simulink model "mseExampleDelayWithLoop"  (R2023b)
settings: Solver=VariableStepAuto  StartTime=0.0  StopTime=10.0  RelTol=1e-3
libraries: simulink x2
settings Model: Creator=DarianMuresan  LastModifiedBy=DarianMuresan

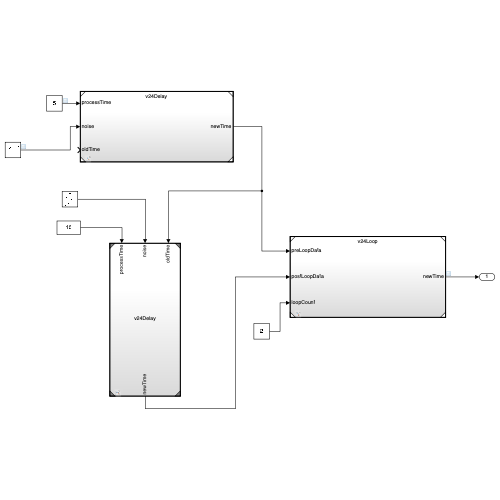
[thumbnail: Simulink's stored preview of the top-level diagram]
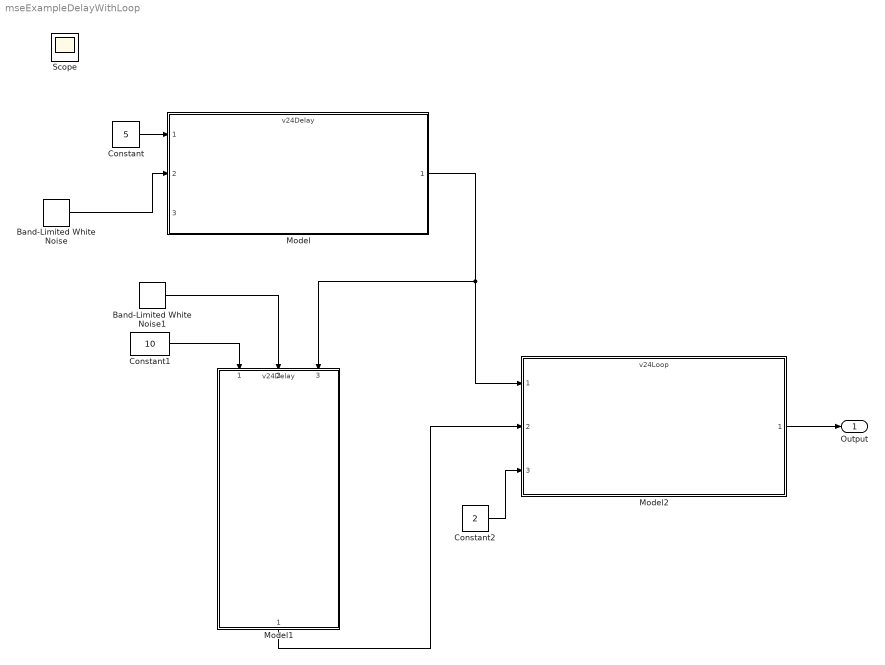
== system mseExampleDelayWithLoop ==
  Band-Limited White Noise : simulink/Sources/Band-Limited White Noise  Cov=[0.01]  Ts=0.1  seed=[23341]
  Band-Limited White Noise1 : simulink/Sources/Band-Limited White Noise  Cov=0.01  Ts=0.1  seed=[23341]
  Constant : Constant  Value=5
  Constant1 : Constant  Value=10
  Constant2 : Constant  Value=2
  Model : ModelReference  ModelNameDialog=v24Delay.slx  SimulationMode=Normal  ModelReferenceVersion=1.6
  Model1 : ModelReference  ModelNameDialog=v24Delay.slx  SimulationMode=Normal  ModelReferenceVersion=1.6
  Model2 : ModelReference  ModelNameDialog=v24Loop.slx  SimulationMode=Normal  ModelReferenceVersion=1.4
  Output : Outport
  Scope : Scope
  wires:
  Constant/1 -> Model/1
  Band-Limited White Noise/1 -> Model/2
  Constant1/1 -> Model1/1
  Band-Limited White Noise1/1 -> Model1/2
  Model/1 -> Model1/3, Model2/1
  Model1/1 -> Model2/2
  Constant2/1 -> Model2/3
  Model2/1 -> Output/1
